simulink model "servo_with_observer_simulink"  (R2021b)
settings: Solver=VariableStepAuto  StartTime=0.0  StopTime=20  RelTol=1e-3
values from neighbouring files (symbols this model uses):
  A = [0, 0, 0, 1, 0, 0 ... (first row only)    [basic_data.m]    (also in basic_data.mat = [0 0 0 0 -22.4688936865 5 0 0 0 6.5 19.3959496459 -3.6 ... (; lqr.mat = [0 0 0 0 -22.4688936865 5 0 0 0 6.5 19.3959496459 -3.6 ... ()
  A_overbar = T*A*inv(T)    [pole_placement.m]    (also in servo.m = [A zeros(6,3);-C zeros(3,3)])
  B = [0, 0 ... (first row only)    [basic_data.m]    (also in basic_data.mat = [0  0; 0  0; 0  0; 27  11.2; 6.06660129535  -1.63757677119; ; lqr.mat = [0  0; 0  0; 0  0; 27  11.2; 6.06660129535  -1.63757677119; )
  B_overbar = T*B    [pole_placement.m]    (also in servo.m = [B;zeros(3,2)])
  C = [1, 0, 0, 0, 0, 0 ... (first row only)    [basic_data.m]    (also in basic_data.mat = [1 0 0 0 1 0 0 0 1 0 0 0 ... (18 elements, 3x6)]; lqr.mat = [1 0 0 0 1 0 0 0 1 0 0 0 ... (18 elements, 3x6)])
  C_overbar = [C,zeros(3,3)]    [servo.m]
  K = real(inv(R)*B'*P)    [ARE.m]    (also in LQR.m = inv(R)*B'*P; Pole_Placement_function.m = h/Wc*S; decoupled.m = F*C_star_star; lqr.mat = [-254.853126299  165.420589601  161.115517614  -14.472900470)
  S = S + co(i)*A^(order+1-i)    [Pole_Placement_function.m]    (also in servo.m = L)
  y_sp = -0.1*C*inv(A)*B*[-0.5+(a-b)/20;0.1+(b-c)/(a+d+10)]    [servo.m]
settings Model: Creator=asus  LastModifiedBy=asus

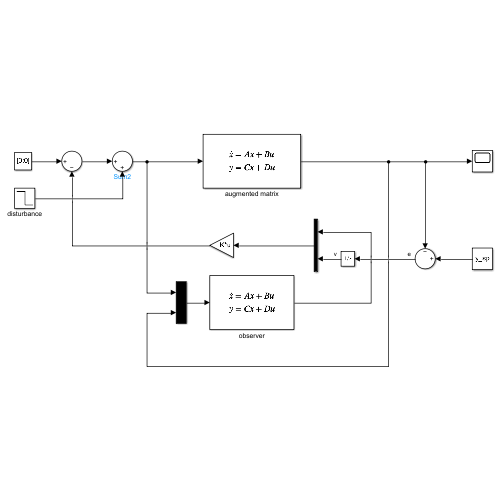
[thumbnail: Simulink's stored preview of the top-level diagram]
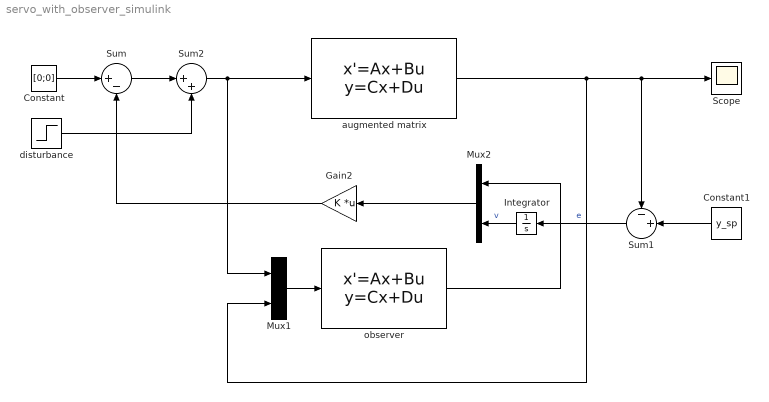
== system servo_with_observer_simulink ==
  Constant : Constant  Value=[0;0]
  Constant1 : Constant  Value=y_sp
  Gain2 : Gain  Gain=K  Multiplication=Matrix(K*u)
  Integrator : Integrator
  Mux1 : Mux  Inputs=2
  Mux2 : Mux  Inputs=2
  Scope : Scope
  Sum : Sum  Inputs=|+-
  Sum1 : Sum  Inputs=-+|
  Sum2 : Sum  Inputs=|++
  augmented matrix : StateSpace  A=A_overbar  B=B_overbar  C=C_overbar  D=zeros(3,2)  InitialCondition=0
  disturbance : Step  Time=10  Before=[0;0]  After=[-1;1]  SampleTime=0
  observer : StateSpace  A=A-S*C  B=[B S]  C=eye(6)  D=zeros(6,5)  InitialCondition=0
  wires:
  Sum2/1 -> Mux1/1, augmented matrix/1
  Mux1/1 -> observer/1
  Constant/1 -> Sum/1
  Gain2/1 -> Sum/2
  Mux2/1 -> Gain2/1
  observer/1 -> Mux2/1
  Constant1/1 -> Sum1/2
  Sum1/1 -> Integrator/1  "e"
  augmented matrix/1 -> Mux1/2, Sum1/1, Scope/1
  Sum/1 -> Sum2/1
  disturbance/1 -> Sum2/2
  Integrator/1 -> Mux2/2  "v"
